simulink model "Ex5"  (Simulink 7.8)
settings: Solver=ode45  StartTime=0.0  StopTime=10.0  RelTol=1e-3
settings Model: Creator=alex  LastModifiedBy=alex

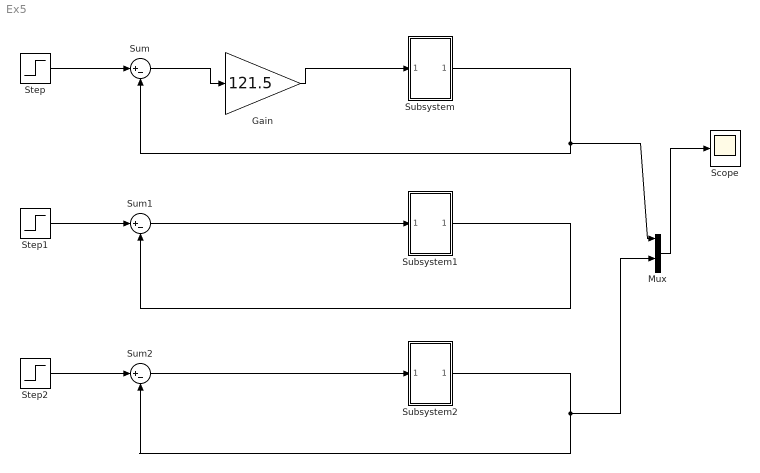
== system Ex5 ==
  Gain : Gain  Gain=121.5
  Mux : Mux
  Scope : Scope
      settings: MaxDataPoints=500000  SampleInput=on
  Step : Step  SampleTime=0
  Step1 : Step  SampleTime=0
  Step2 : Step  SampleTime=0
  Subsystem : Subsystem
  Subsystem1 : Subsystem
  Subsystem2 : Subsystem
  Sum : Sum  Inputs=|+-
  Sum1 : Sum  Inputs=|+-
  Sum2 : Sum  Inputs=|+-
  wires:
  Subsystem/1(Out1) -> Sum/2, Mux/1
  Step/1 -> Sum/1
  Sum/1 -> Gain/1
  Gain/1 -> Subsystem/1(In1)
  Mux/1 -> Scope/1
  Subsystem1/1(Out1) -> Sum1/2
  Step1/1 -> Sum1/1
  Subsystem2/1(Out1) -> Sum2/2, Mux/3
  Step2/1 -> Sum2/1
  Sum2/1 -> Subsystem2/1(In1)
  Sum1/1 -> Subsystem1/1(In1)

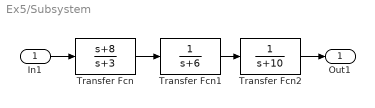
== system Ex5/Subsystem ==
  In1 : Inport
  Transfer Fcn : TransferFcn  Numerator=[1 8]  Denominator=[1 3]
  Transfer Fcn1 : TransferFcn  Denominator=[1 6]
  Transfer Fcn2 : TransferFcn  Denominator=[1 10]
  Out1 : Outport
  wires:
  Transfer Fcn1/1 -> Transfer Fcn2/1
  Transfer Fcn/1 -> Transfer Fcn1/1
  In1/1 -> Transfer Fcn/1
  Transfer Fcn2/1 -> Out1/1

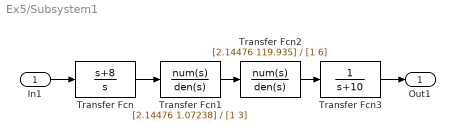
== system Ex5/Subsystem1 ==
  In1 : Inport
  Transfer Fcn : TransferFcn  Numerator=[1 8]  Denominator=[1 0]
  Transfer Fcn1 : TransferFcn  Numerator=[2.14476 1.07238]  Denominator=[1 3]
  Transfer Fcn2 : TransferFcn  Numerator=[2.14476 119.935]  Denominator=[1 6]
  Transfer Fcn3 : TransferFcn  Denominator=[1 10]
  Out1 : Outport
  wires:
  Transfer Fcn1/1 -> Transfer Fcn2/1
  Transfer Fcn/1 -> Transfer Fcn1/1
  In1/1 -> Transfer Fcn/1
  Transfer Fcn2/1 -> Transfer Fcn3/1
  Transfer Fcn3/1 -> Out1/1

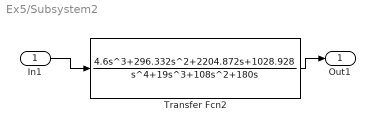
== system Ex5/Subsystem2 ==
  In1 : Inport
  Transfer Fcn2 : TransferFcn  Numerator=[4.6 296.332 2204.872 1028.928]  Denominator=[1 19 108 180 0]
  Out1 : Outport
  wires:
  In1/1 -> Transfer Fcn2/1
  Transfer Fcn2/1 -> Out1/1
